simulink model "q1LinearModel"  (R2019a)
settings: Solver=VariableStepAuto  StartTime=0.0  StopTime=1000  RelTol=1e-3
values from neighbouring files (symbols this model uses):
  Ka = 4.3    [q1.m]
  m = 1230    [q1.m]
  Vnom = 40/3.6    (= 11.1111111111)    [q1.m]
  Vw = 5    [q1.m]
libraries: cstblocks x4
settings Model: Creator=Nir Lalum  LastModifiedBy=Nir Lalum

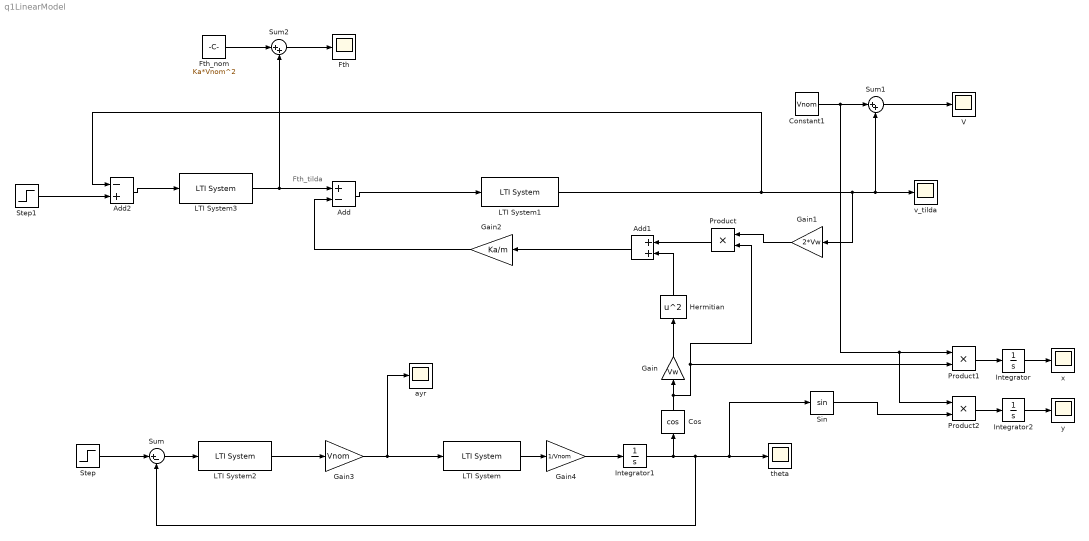
== system q1LinearModel ==
  note: Fth_tilda
  Add : Sum  Inputs=+-
  Add1 : Sum
  Add2 : Sum  Inputs=-+
  Constant1 : Constant  Value=Vnom
  Cos : Trigonometry  Operator=cos
  "Fth " : Scope
  Fth_nom : Constant  Value=Ka*Vnom^2
  Gain : Gain  Gain=Vw
  Gain1 : Gain  Gain=2*Vw
  Gain2 : Gain  Gain=Ka/m
  Gain3 : Gain  Gain=Vnom
  Gain4 : Gain  Gain=1/Vnom
  Hermitian : Math  Operator=square  SaturateOnIntegerOverflow=on
  Integrator : Integrator
  Integrator1 : Integrator
  Integrator2 : Integrator
  LTI System : cstblocks/LTI System  sys=G_ayr_ay  IC=[]
  LTI System1 : cstblocks/LTI System  sys=P_v  IC=[]
  LTI System2 : cstblocks/LTI System  sys=C_theta_tilda  IC=[]
  LTI System3 : cstblocks/LTI System  sys=C_v  IC=[]
  Product : Product
  Product1 : Product
  Product2 : Product
  Sin : Trigonometry
  Step : Step  Time=50  After=pi  SampleTime=0
  Step1 : Step  Time=0  After=10/3.6  SampleTime=0
  Sum : Sum  Inputs=|+-
  Sum1 : Sum  Inputs=|++
  Sum2 : Sum  Inputs=|++
  V : Scope
  ayr : Scope
  theta : Scope
  v_tilda : Scope
  x : Scope
  y : Scope
  wires:
  LTI System/1 -> Gain4/1
  Integrator1/1 -> Sum/2, Sin/1, theta/1, Cos/1
  Gain/1 -> Hermitian/1
  Hermitian/1 -> Add1/2
  Add1/1 -> Gain2/1
  LTI System3/1 -> Add/1, Sum2/2
  Cos/1 -> Product1/2, Product/2, Gain/1
  Gain1/1 -> Product/1
  Product/1 -> Add1/1
  Add/1 -> LTI System1/1
  Gain2/1 -> Add/2
  LTI System2/1 -> Gain3/1
  Sum/1 -> LTI System2/1
  Step/1 -> Sum/1
  Add2/1 -> LTI System3/1
  Step1/1 -> Add2/2
  LTI System1/1 -> Gain1/1, Sum1/2, v_tilda/1, Add2/1
  Constant1/1 -> Product2/1, Product1/1, Sum1/1
  Sum1/1 -> V/1
  Gain3/1 -> ayr/1, LTI System/1
  Gain4/1 -> Integrator1/1
  Fth_nom/1 -> Sum2/1
  Sum2/1 -> "Fth "/1
  Sin/1 -> Product2/2
  Product1/1 -> Integrator/1
  Product2/1 -> Integrator2/1
  Integrator/1 -> x/1
  Integrator2/1 -> y/1
